simulink model "property_3_unsafe_test"  (Simulink 8.5)
settings: Solver=VariableStepDiscrete  StartTime=0.0  StopTime=10.0  RelTol=1e-3
settings Model: Creator=arnaud  LastModifiedBy=teme  CovSFcnEnable=off
settings DataIOCC: SaveFormat=Structure
settings DebuggingCC: SolverPrmCheckMsg=warning  FcnCallInpInsideContextMsg=UseLocalSettings

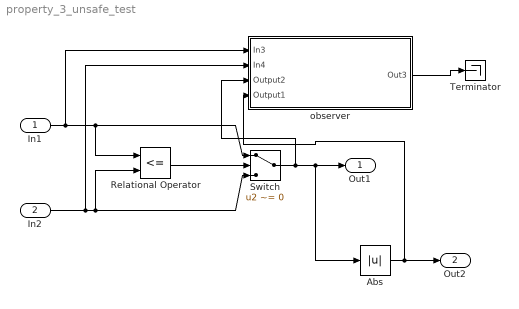
== system property_3_unsafe_test ==
  In1 : Inport
  In2 : Inport  Port=2
  Abs : Abs
  Relational Operator : RelationalOperator  Operator=<=  OutDataTypeStr=boolean
  Switch : Switch  Criteria=u2 ~= 0
  Terminator : Terminator
  observer : Subsystem  TreatAsAtomicUnit=on  mask(Observer){AnnotationType=ensures, ObserverType=ellipsoid}
      mask prompts: AnnotationType "Type of annotation (pre/post...)"; ObserverType "Observer type"
      mask help:
      | Set an observer for the system.
      | The annotation type parameter sets the type of observer:
      | - requires : pre-condition
      | - ensures : post-condition
      | - assert : an assertion
      | - observer : the observer computes a special type of properties
      mask TypeOptions AnnotationType: ensures | requires | assert | observer
      mask Callback AnnotationType:
      | paramStr = get_param(gcb, 'MaskValues');
      | 
      | if strcmp(paramStr{1}(1),'o')
      |     set_param(gcb,'MaskVisibilities',{'on';'on'});
      |     paramStr{2} = 'ellipsoid';
      |     set_param(gcb,'MaskValues',paramStr);
      | else
      |     set_param(gcb,'MaskVisibilities',{'on';'off'});
      | end
      mask Callback ObserverType:
      | paramStr = get_param(gcb, 'MaskValues');
      | 
      | if strcmp(paramStr{1}(1),'observer')
      |     set_param(gcb,'MaskVisibilities',{'on';'on'});
      |     paramStr{2} = 'ellipsoid';
      |     set_param(gcb,'MaskValues',paramStr);
      | else
      |     set_param(gcb,'MaskVisibilities',{'on';'off'});
      | end
      mask Display:
      | color('red');
      | text(0.5, 0.5, 'Observer Block', 'horizontalAlignment', 'center');
  Out1 : Outport
  Out2 : Outport  Port=2
  wires:
  In1/1 -> observer/1(In3), Relational Operator/1, Switch/1
  In2/1 -> observer/2(In4), Relational Operator/2, Switch/3
  Relational Operator/1 -> Switch/2
  observer/1(Out3) -> Terminator/1
  Switch/1 -> observer/3(Output2), Out1/1, Abs/1
  Abs/1 -> observer/4(Output1), Out2/1

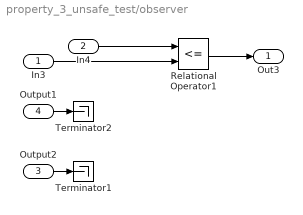
== system property_3_unsafe_test/observer ==
  In3 : Inport
  In4 : Inport  Port=2
  Output2 : Inport  Port=3
  Output1 : Inport  Port=4
  Relational Operator1 : RelationalOperator  Operator=<=  OutDataTypeStr=boolean
  Terminator1 : Terminator
  Terminator2 : Terminator
  Out3 : Outport
  wires:
  In3/1 -> Relational Operator1/2
  Output2/1 -> Terminator1/1
  Relational Operator1/1 -> Out3/1
  In4/1 -> Relational Operator1/1
  Output1/1 -> Terminator2/1
